simulink model "EarlyReturn3_2018a"  (R2020a)
settings: Solver=VariableStepAuto  StartTime=0.0  StopTime=10.0  RelTol=1e-3
settings Model: Creator=apple  LastModifiedBy=apple

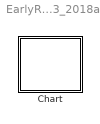
== system EarlyReturn3_2018a ==
  Chart : Stateflow chart  TreatAsAtomicUnit=on

== stateflow chart EarlyReturn3_2018a/Chart ==
  state A
    en: fprintf("en_A")
    ex: fprintf("ex_A")
  state B
    en: fprintf("en_B")
    ex: fprintf("ex_B")
  state C
    en: fprintf("en_C")
    ex: fprintf("ex_C")
  (default) -> A : {data=1;}
  A -> B [order 1] : [data==1]{data=2;E}
  A -> C [order 2] : E
  data: data local int32
  events: E local FUNCTION_CALL_EVENT
